simulink model "hw4_tank_PP"  (R2023b)
settings: Solver=ode45  StartTime=0.0  StopTime=50  FixedStep=0.000001  RelTol=1e-3
values from neighbouring files (symbols this model uses):
  A = 1    [Copy_of_hw1_four_channel_bilateral_teleoperation_params.m]    (also in hw1_four_channel_bilateral_teleoperation_params.m; hw2_2_3_channel_bilateral_teleoperation_params.m; hw3_scattering_teleop_FP_params.m = 1.5; hw3_scattering_teleop_PP_params.m)
  Ak = [1 Ts ... (first row only)    [hw3_scattering_teleop_FP_params.m]    (also in hw3_scattering_teleop_PP_params.m; hw4_tank_FP_params.m; hw4_tank_PP_params.m; no_noise_hw4_tank_PP_params.m)
  B = [Ts^2/2; Ts]    [hw3_scattering_teleop_FP_params.m]    (also in hw3_scattering_teleop_PP_params.m; hw4_tank_FP_params.m; hw4_tank_PP_params.m; no_noise_hw4_tank_PP_params.m)
  Be = 100    [Copy_of_hw1_four_channel_bilateral_teleoperation_params.m]    (also in hw1_four_channel_bilateral_teleoperation_params.m; hw2_2_3_channel_bilateral_teleoperation_params.m; hw3_scattering_teleop_FP_params.m; hw3_scattering_teleop_PP_params.m)
  beta = 0.1    [hw4_tank_FP_params.m]    (also in hw4_tank_PP_params.m; no_noise_hw4_tank_PP_params.m; test_no_noise_hw4_tank_PP_params.m)
  Bh = 1    [Copy_of_hw1_four_channel_bilateral_teleoperation_params.m]    (also in hw1_four_channel_bilateral_teleoperation_params.m; hw2_2_3_channel_bilateral_teleoperation_params.m; hw3_scattering_teleop_FP_params.m; hw3_scattering_teleop_PP_params.m)
  Bm = 20*0.8    (= 16)    [Copy_of_hw1_four_channel_bilateral_teleoperation_params.m]    (also in hw1_four_channel_bilateral_teleoperation_params.m; hw2_2_3_channel_bilateral_teleoperation_params.m; hw3_scattering_teleop_FP_params.m; hw3_scattering_teleop_PP_params.m)
  Bs = 4*Bm    (= 64)    [Copy_of_hw1_four_channel_bilateral_teleoperation_params.m]    (also in hw1_four_channel_bilateral_teleoperation_params.m; hw2_2_3_channel_bilateral_teleoperation_params.m; hw3_scattering_teleop_FP_params.m; hw3_scattering_teleop_PP_params.m)
  C = [1 0]    [hw3_scattering_teleop_FP_params.m]    (also in hw3_scattering_teleop_PP_params.m; hw4_tank_FP_params.m; hw4_tank_PP_params.m; no_noise_hw4_tank_PP_params.m)
  d = 1    [hw2_2_3_channel_bilateral_teleoperation_params.m]    (also in hw3_scattering_teleop_FP_params.m = 10; hw3_scattering_teleop_PP_params.m = 10; hw4_tank_FP_params.m = 10; hw4_tank_PP_params.m = 10)
  Dh = 20*0.8    (= 16)    [Copy_of_hw1_four_channel_bilateral_teleoperation_params.m]    (also in hw1_four_channel_bilateral_teleoperation_params.m; hw2_2_3_channel_bilateral_teleoperation_params.m; hw3_scattering_teleop_FP_params.m; hw3_scattering_teleop_PP_params.m)
  Dm = 5    [Copy_of_hw1_four_channel_bilateral_teleoperation_params.m]    (also in hw1_four_channel_bilateral_teleoperation_params.m; hw2_2_3_channel_bilateral_teleoperation_params.m; hw3_scattering_teleop_FP_params.m; hw3_scattering_teleop_PP_params.m = 0)
  Ds = 10    [Copy_of_hw1_four_channel_bilateral_teleoperation_params.m]    (also in hw1_four_channel_bilateral_teleoperation_params.m; hw2_2_3_channel_bilateral_teleoperation_params.m; hw3_scattering_teleop_FP_params.m = 0; hw3_scattering_teleop_PP_params.m = 0)
  Fc = 1    [Copy_of_hw1_four_channel_bilateral_teleoperation_params.m]    (also in hw1_four_channel_bilateral_teleoperation_params.m; hw2_2_3_channel_bilateral_teleoperation_params.m; hw3_scattering_teleop_FP_params.m; hw3_scattering_teleop_PP_params.m)
  Flp = 0.5    [Copy_of_hw1_four_channel_bilateral_teleoperation_params.m]    (also in hw1_four_channel_bilateral_teleoperation_params.m; hw2_2_3_channel_bilateral_teleoperation_params.m; hw3_scattering_teleop_FP_params.m = 0.01; hw3_scattering_teleop_PP_params.m = 0.01)
  Flp1 = 0.5    [hw3_scattering_teleop_FP_params.m]    (also in hw3_scattering_teleop_PP_params.m; hw4_tank_FP_params.m; hw4_tank_PP_params.m; no_noise_hw4_tank_PP_params.m)
  Hd = 1    [hw4_tank_FP_params.m]    (also in hw4_tank_PP_params.m; no_noise_hw4_tank_PP_params.m; test_no_noise_hw4_tank_PP_params.m)
  Hm_init = 5    [hw4_tank_FP_params.m]    (also in hw4_tank_PP_params.m; no_noise_hw4_tank_PP_params.m; test_no_noise_hw4_tank_PP_params.m = 0)
  Hs_init = 5    [hw4_tank_FP_params.m]    (also in hw4_tank_PP_params.m; no_noise_hw4_tank_PP_params.m; test_no_noise_hw4_tank_PP_params.m = 0)
  Jh = 1    [Copy_of_hw1_four_channel_bilateral_teleoperation_params.m]    (also in hw1_four_channel_bilateral_teleoperation_params.m; hw2_2_3_channel_bilateral_teleoperation_params.m; hw3_scattering_teleop_FP_params.m; hw3_scattering_teleop_PP_params.m)
  Ke = 200    [Copy_of_hw1_four_channel_bilateral_teleoperation_params.m]    (also in hw1_four_channel_bilateral_teleoperation_params.m; hw2_2_3_channel_bilateral_teleoperation_params.m; hw3_scattering_teleop_FP_params.m; hw3_scattering_teleop_PP_params.m)
  Km = 10*1    (= 10)    [Copy_of_hw1_four_channel_bilateral_teleoperation_params.m]    (also in hw1_four_channel_bilateral_teleoperation_params.m; hw2_2_3_channel_bilateral_teleoperation_params.m; hw3_scattering_teleop_FP_params.m; hw3_scattering_teleop_PP_params.m)
  Ks = 4*Km    (= 40)    [Copy_of_hw1_four_channel_bilateral_teleoperation_params.m]    (also in hw1_four_channel_bilateral_teleoperation_params.m; hw2_2_3_channel_bilateral_teleoperation_params.m; hw3_scattering_teleop_FP_params.m; hw3_scattering_teleop_PP_params.m)
  Mm = 0.5    [Copy_of_hw1_four_channel_bilateral_teleoperation_params.m]    (also in hw1_four_channel_bilateral_teleoperation_params.m; hw2_2_3_channel_bilateral_teleoperation_params.m; hw3_scattering_teleop_FP_params.m; hw3_scattering_teleop_PP_params.m)
  Ms = 2    [Copy_of_hw1_four_channel_bilateral_teleoperation_params.m]    (also in hw1_four_channel_bilateral_teleoperation_params.m; hw2_2_3_channel_bilateral_teleoperation_params.m; hw3_scattering_teleop_FP_params.m; hw3_scattering_teleop_PP_params.m)
  noise = 0.001    [hw3_scattering_teleop_FP_params.m]    (also in hw3_scattering_teleop_PP_params.m; hw4_tank_FP_params.m = 0.0001; hw4_tank_PP_params.m; no_noise_hw4_tank_PP_params.m)
  Ph = 10*1    (= 10)    [Copy_of_hw1_four_channel_bilateral_teleoperation_params.m]    (also in hw1_four_channel_bilateral_teleoperation_params.m; hw2_2_3_channel_bilateral_teleoperation_params.m; hw3_scattering_teleop_FP_params.m; hw3_scattering_teleop_PP_params.m)
  R = 1    [hw3_scattering_teleop_FP_params.m]    (also in hw3_scattering_teleop_PP_params.m; hw4_tank_FP_params.m; hw4_tank_PP_params.m; no_noise_hw4_tank_PP_params.m)
  tlcAlpha = 2    [hw4_tank_FP_params.m]    (also in hw4_tank_PP_params.m; no_noise_hw4_tank_PP_params.m; test_no_noise_hw4_tank_PP_params.m)
  Ts = 0.001    [hw3_scattering_teleop_FP_params.m]    (also in hw3_scattering_teleop_PP_params.m; hw4_tank_FP_params.m; hw4_tank_PP_params.m; no_noise_hw4_tank_PP_params.m)
  x0 = [0 0]    [hw3_scattering_teleop_FP_params.m]    (also in hw3_scattering_teleop_PP_params.m; hw4_tank_FP_params.m; hw4_tank_PP_params.m; no_noise_hw4_tank_PP_params.m)
  xe = 5    [Copy_of_hw1_four_channel_bilateral_teleoperation_params.m]    (also in hw1_four_channel_bilateral_teleoperation_params.m = 0.8; hw2_2_3_channel_bilateral_teleoperation_params.m = 2; hw3_scattering_teleop_FP_params.m = 0.8; hw3_scattering_teleop_PP_params.m = 2)
undefined symbols (not defined in the file or in its folder): Discrete, Time
libraries: simulink x3, ctrlSharedLib x2, cstblocks x1
settings Model: Creator=86180  LastModifiedBy=86180

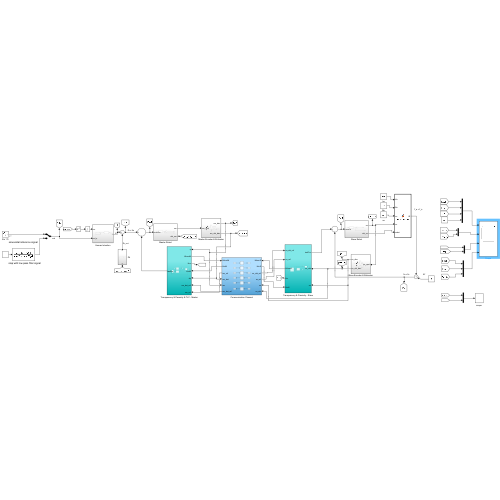
[thumbnail: Simulink's stored preview of the top-level diagram]
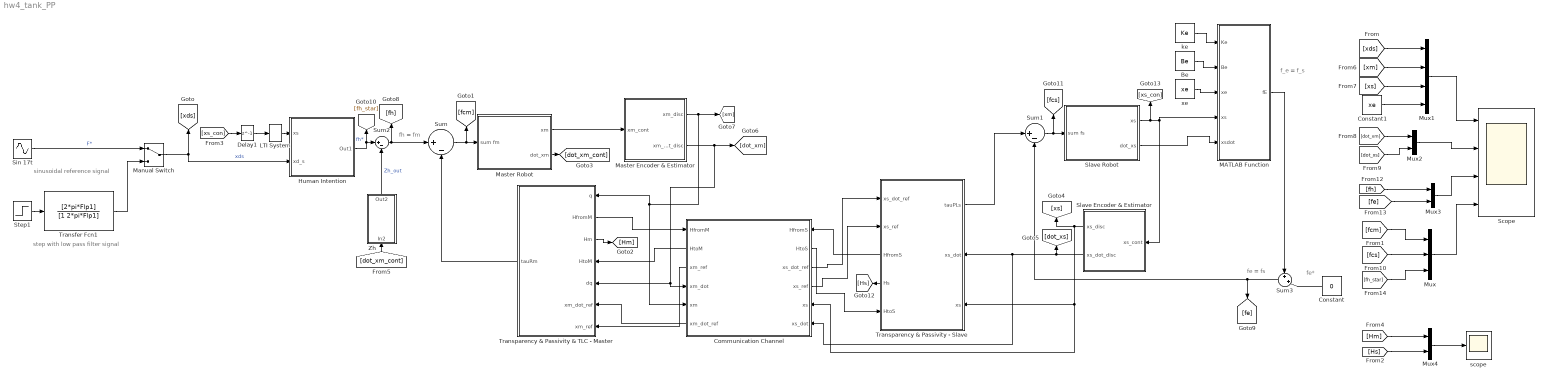
== system hw4_tank_PP ==
  note: f_e = f_s
  note: fe*
  note: fe = fs
  note: fh = fm
  note: sinusoidal reference signal
  note: step with low pass filter signal
  Be : Constant  Value=Be
  Communication Channel : Subsystem
      settings: PortSchema="{\"entries\":[{\"content\":{\"sides\":[{\"content\":{\"connectorIds\":[\"In1\",\"Out4\",\"Out5\",\"Out6\",\"In2\",\"In3\"]},\"type\":\"ConnectorPlacement.EquallySpacedRectSide\",\"uuid\":\"1c070cf8-9aa7-4f7b-8e2f-2632c2893f69\"},{\"content\":{\"connectorIds\":[\"In4\",\"Out1\",\"Out2\",\"In5\",\"In6\",\"Out3\"],\"side\":\"RIGHT\"},\"type\":\"ConnectorPlacement.EquallySpacedRectSide\",\"uuid\":\"32173565-3523-4dfc-9820-763c87098354\"},{\"content\":{\"side\":\"TOP\"},\"type\":\"ConnectorPlacement.EquallySpacedRectSide\",\"uuid\":\"13187df6-bf6f-436e-a2ee-34150977e6a8\"},{\"content\":{\"side\":\"HIDDEN\"},\"type\":\"ConnectorPlacement.EquallySpacedRectSide\",\"uuid\":\"1e5bcdd7-6028-40f7-b524-727817e519ff\"}]},\"type\":\"ConnectorPlacement.EquallySpacedConnector\",\"uuid\":\"c84d0440-83b9-4b92-a10a-1f72bb115b54\"}],\"packageUris\":[\"http://schema.mathworks.com/mf0/Connector/R2020b\"],\"version\":\"1.0\"}"
  Constant : Constant  Value=0
  Constant1 : Constant  Value=xe
  Delay1 : Delay  DelayLength=1  SampleTime=Ts
  Human Intention : Subsystem
  LTI System : cstblocks/LTI System  sys=1  IC=[]  PadeOrder=0
  MATLAB Function : MATLAB Function  TreatAsAtomicUnit=on
  Manual Switch : ManualSwitch
  Master Encoder & Estimator : Subsystem
  Master Robot : Subsystem
  Mux : Mux  Inputs=3
  Mux1 : Mux
  Mux2 : Mux  Inputs=2
  Mux3 : Mux  Inputs=2
  Mux4 : Mux  Inputs=2
  Scope : Scope  NumInputPorts=4
  Sin 17t : Sin  Amplitude=A  Frequency=Fc  SampleTime=0
  Slave Encoder & Estimator : Subsystem
  Slave Robot : Subsystem
  Step1 : Step  Time=0.5  After=A  SampleTime=0
  Sum : Sum  Inputs=|+-
  Sum1 : Sum  Inputs=|+-
  Sum2 : Sum  Inputs=|+-
  Sum3 : Sum  Inputs=+|+|
  Transfer Fcn1 : TransferFcn  Numerator=[2*pi*Flp1]  Denominator=[1 2*pi*Flp1]
  Transparency & Passivity & TLC - Master : Subsystem
      settings: PortSchema="{\"entries\":[{\"content\":{\"sides\":[{\"content\":{\"connectorIds\":[\"In1\",\"Out2\",\"Out3\",\"In2\",\"In3\",\"In4\",\"In5\"]},\"type\":\"ConnectorPlacement.EquallySpacedRectSide\",\"uuid\":\"254acbc8-8c2d-438f-adc1-7e75d47258bf\"},{\"content\":{\"connectorIds\":[\"Out1\"],\"side\":\"RIGHT\"},\"type\":\"ConnectorPlacement.EquallySpacedRectSide\",\"uuid\":\"ebc7579d-fe16-4fae-be7d-b1631322842e\"},{\"content\":{\"side\":\"TOP\"},\"type\":\"ConnectorPlacement.EquallySpacedRectSide\",\"uuid\":\"d0c6f2f9-df1e-40c2-885e-c029821bef96\"}]},\"type\":\"ConnectorPlacement.EquallySpacedConnector\",\"uuid\":\"8dee1f1f-c5e6-463a-a0e9-fbee882b1e3c\"}],\"packageUris\":[\"http://schema.mathworks.com/mf0/Connector/R2020b\"],\"version\":\"1.0\"}"
  Transparency & Passivity - Slave : Subsystem
      settings: PortSchema="{\"entries\":[{\"content\":{\"sides\":[{\"content\":{\"connectorIds\":[\"In1\",\"In2\",\"Out2\",\"Out3\",\"In3\"]},\"type\":\"ConnectorPlacement.EquallySpacedRectSide\",\"uuid\":\"bd42ff73-50dc-42d6-9dfb-d60369543bc9\"},{\"content\":{\"connectorIds\":[\"Out1\",\"In4\",\"In5\"],\"side\":\"RIGHT\"},\"type\":\"ConnectorPlacement.EquallySpacedRectSide\",\"uuid\":\"78e50b8f-eeac-432c-8eb4-27f06d4ce9eb\"},{\"content\":{\"side\":\"TOP\"},\"type\":\"ConnectorPlacement.EquallySpacedRectSide\",\"uuid\":\"9e8e9e88-d3ad-4c46-818b-4ad777acb646\"}]},\"type\":\"ConnectorPlacement.EquallySpacedConnector\",\"uuid\":\"6c4e05d2-6c15-4cd7-9da0-0c4b09a4ecbf\"}],\"packageUris\":[\"http://schema.mathworks.com/mf0/Connector/R2020b\"],\"version\":\"1.0\"}"
  Zh : Subsystem
  ke : Constant  Value=Ke
  scope : Scope
  xe : Constant  Value=xe
  wires:
  Manual Switch/1 -> Human Intention/2(xd_s), [xds]  "xds"
  Zh/1(Out2) -> Sum2/2  "Zh_out"
  Transfer Fcn1/1 -> Manual Switch/2
  Human Intention/1(Out1) -> [fh_star], Sum2/1  "fh*"
  Sin 17t/1 -> Manual Switch/1  "F*"
  Step1/1 -> Transfer Fcn1/1
  ke/1 -> MATLAB Function/1(Ke)
  xe/1 -> MATLAB Function/3(xe)
  Slave Robot/1(xs) -> MATLAB Function/4(xs), Slave Encoder & Estimator/1(xs_cont), [xs_con]
  MATLAB Function/1(fE) -> Sum3/1
  Be/1 -> MATLAB Function/2(Be)
  Sum2/1 -> Sum/1, [fh]
  Slave Robot/2(dot_xs) -> MATLAB Function/5(xsdot)
  Sum3/1 -> Sum1/2, [fe]
  Constant/1 -> Sum3/2
  [xds] -> Mux1/1
  Sum/1 -> [fcm], Master Robot/1(sum fm)
  [dot_xm_cont] -> Zh/1(In2)
  [xm] -> Mux1/2
  [xs] -> Mux1/3
  [dot_xm] -> Mux2/1
  Sum1/1 -> [fcs], Slave Robot/1(sum fs)
  [fh] -> Mux3/1
  [fe] -> Mux3/2
  [fh_star] -> Mux/3
  [fcs] -> Mux/2
  [fcm] -> Mux/1
  Constant1/1 -> Mux1/4
  [dot_xs] -> Mux2/2
  Mux1/1 -> Scope/1
  Mux2/1 -> Scope/2
  Mux3/1 -> Scope/3
  Mux/1 -> Scope/4
  [xs_con] -> Delay1/1
  Master Robot/1(xm) -> Master Encoder & Estimator/1(xm_cont)
  Master Encoder & Estimator/1(xm_disc) -> Communication Channel/6(xm), Transparency & Passivity & TLC - Master/1(q), [xm]
  Master Encoder & Estimator/2(xm_dot_disc) -> Communication Channel/5(xm_dot), Transparency & Passivity & TLC - Master/3(dq), [dot_xm]
  Slave Encoder & Estimator/2(xs_dot_disc) -> Communication Channel/3(xs_dot), Transparency & Passivity - Slave/4(xs_dot), [dot_xs]
  Slave Encoder & Estimator/1(xs_disc) -> Communication Channel/2(xs), Transparency & Passivity - Slave/5(xs), [xs]
  Delay1/1 -> LTI System/1
  LTI System/1 -> Human Intention/1(xs)
  Master Robot/2(dot_xm) -> [dot_xm_cont]
  Transparency & Passivity & TLC - Master/2(HfromM) -> Communication Channel/4(HfromM)
  Transparency & Passivity & TLC - Master/1(tauRm) -> Sum/2
  Communication Channel/1(HtoM) -> Transparency & Passivity & TLC - Master/2(HtoM)
  Transparency & Passivity - Slave/2(HfromS) -> Communication Channel/1(HfromS)
  Transparency & Passivity - Slave/1(tauPLs) -> Sum1/1
  Communication Channel/4(HtoS) -> Transparency & Passivity - Slave/3(HtoS)
  Communication Channel/5(xs_dot_ref) -> Transparency & Passivity - Slave/1(xs_dot_ref)
  Communication Channel/6(xs_ref) -> Transparency & Passivity - Slave/2(xs_ref)
  [Hm] -> Mux4/1
  [Hs] -> Mux4/2
  Mux4/1 -> scope/1
  Transparency & Passivity & TLC - Master/3(Hm) -> [Hm]
  Transparency & Passivity - Slave/3(Hs) -> [Hs]
  Communication Channel/2(xm_ref) -> Transparency & Passivity & TLC - Master/5(xm_ref)
  Communication Channel/3(xm_dot_ref) -> Transparency & Passivity & TLC - Master/4(xm_dot_ref)

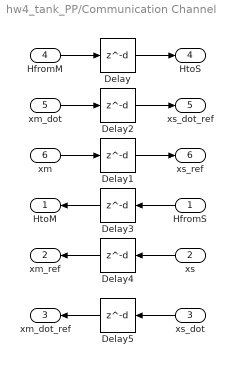
== system hw4_tank_PP/Communication Channel ==
  HfromS : Inport
  xs : Inport  Port=2
  xs_dot : Inport  Port=3
  HfromM : Inport  Port=4
  xm_dot : Inport  Port=5
  xm : Inport  Port=6
  Delay{,1..5} (6 alike) : Delay  DelayLength=d  SampleTime=Ts
  HtoM : Outport
  xm_ref : Outport  Port=2
  xm_dot_ref : Outport  Port=3
  HtoS : Outport  Port=4
  xs_dot_ref : Outport  Port=5
  xs_ref : Outport  Port=6
  wires:
  HfromS/1 -> Delay3/1
  xm_dot/1 -> Delay2/1
  xs/1 -> Delay4/1
  Delay4/1 -> xm_ref/1
  xm/1 -> Delay1/1
  Delay1/1 -> xs_ref/1
  Delay2/1 -> xs_dot_ref/1
  HfromM/1 -> Delay/1
  Delay/1 -> HtoS/1
  Delay3/1 -> HtoM/1
  Delay5/1 -> xm_dot_ref/1
  xs_dot/1 -> Delay5/1

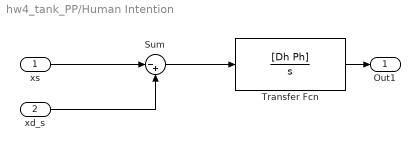
== system hw4_tank_PP/Human Intention ==
  xs : Inport
  xd_s : Inport  Port=2
  Sum : Sum  Inputs=|-+
  Transfer Fcn : TransferFcn  Numerator=[Dh Ph]  Denominator=[1 0]
  Out1 : Outport
  wires:
  Sum/1 -> Transfer Fcn/1
  xd_s/1 -> Sum/2
  xs/1 -> Sum/1
  Transfer Fcn/1 -> Out1/1

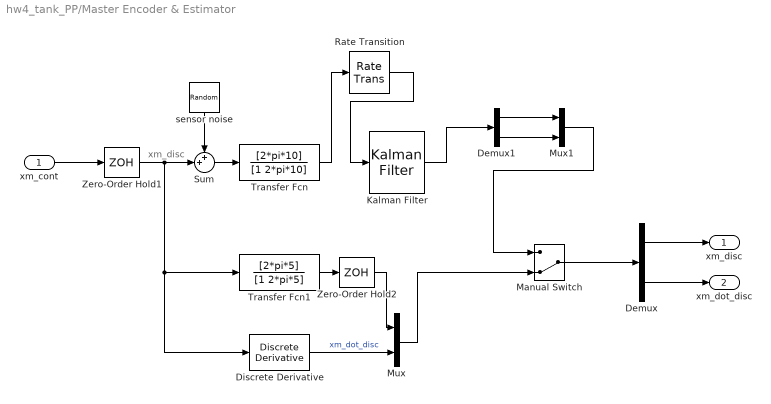
== system hw4_tank_PP/Master Encoder & Estimator ==
  note: xm_disc
  xm_cont : Inport
  Demux : Demux  Outputs=2
  Demux1 : Demux  Outputs=2
  Discrete Derivative : simulink/Discrete/Discrete Derivative  gainval=1.0  ICPrevScaledInput=0.0  OutMin=[]  OutMax=[]  OutDataType=fixdt(1, 16)  OutScaling=2^-10  DoSatur=off
  Kalman Filter : ctrlSharedLib/Kalman Filter  TimeDomain=Discrete-Time  UseCurrentEstimator=on  ModelSource=Individual A, B, C, D matrices  ModelSourceVariable=ss(0.95,1,1,0,1)  A=Ak  B=B  C=C  D=0  NumberOfStates=2  NumberOfInputs=1  NumberOfOutputs=1  InitialEstimateSource=Dialog  X0=x0  P0=10  UseK=off  UseGH=off  NumberOfProcessNoiseInputs=1  G=1  TimeInvariantG=on  H=0  TimeInvariantH=on  Q=Q_m  TimeInvariantQ=on  R=R  TimeInvariantR=on  N=0  TimeInvariantN=on  AddInputPort=off  AddEnablePort=off  OutputEstimatedY=off  OutputP=off  Ts=Ts
  Manual Switch : ManualSwitch  CurrentSetting=0
  Mux : Mux  Inputs=2
  Mux1 : Mux  Inputs=2
  Rate Transition : RateTransition
  Sum : Sum  Inputs=++|
  Transfer Fcn : TransferFcn  Numerator=[2*pi*10]  Denominator=[1 2*pi*10]
  Transfer Fcn1 : TransferFcn  Numerator=[2*pi*5]  Denominator=[1 2*pi*5]
  Zero-Order Hold1 : ZeroOrderHold  SampleTime=Ts
  Zero-Order Hold2 : ZeroOrderHold  SampleTime=Ts
  sensor noise : RandomNumber  Variance=noise  SampleTime=Ts
  xm_disc : Outport
  xm_dot_disc : Outport  Port=2
  wires:
  Demux/2 -> xm_dot_disc/1
  Discrete Derivative/1 -> Mux/2  "xm_dot_disc"
  Manual Switch/1 -> Demux/1
  Zero-Order Hold1/1 -> Discrete Derivative/1, Transfer Fcn1/1, Sum/2
  xm_cont/1 -> Zero-Order Hold1/1
  Demux/1 -> xm_disc/1
  sensor noise/1 -> Sum/1
  Mux/1 -> Manual Switch/2
  Mux1/1 -> Manual Switch/1
  Sum/1 -> Transfer Fcn/1
  Kalman Filter/1 -> Demux1/1
  Demux1/1 -> Mux1/1
  Demux1/2 -> Mux1/2
  Transfer Fcn/1 -> Rate Transition/1
  Rate Transition/1 -> Kalman Filter/1
  Transfer Fcn1/1 -> Zero-Order Hold2/1
  Zero-Order Hold2/1 -> Mux/1

== system hw4_tank_PP/Master Robot ==
  note: dot_xm
  note: xm
      | xm
  sum fm : Inport
  Integrator1 : Integrator
  Transfer Fcn : TransferFcn  Denominator=[Mm Dm]
  xm : Outport
  dot_xm : Outport  Port=2
  wires:
  Integrator1/1 -> xm/1
  Transfer Fcn/1 -> dot_xm/1, Integrator1/1
  sum fm/1 -> Transfer Fcn/1

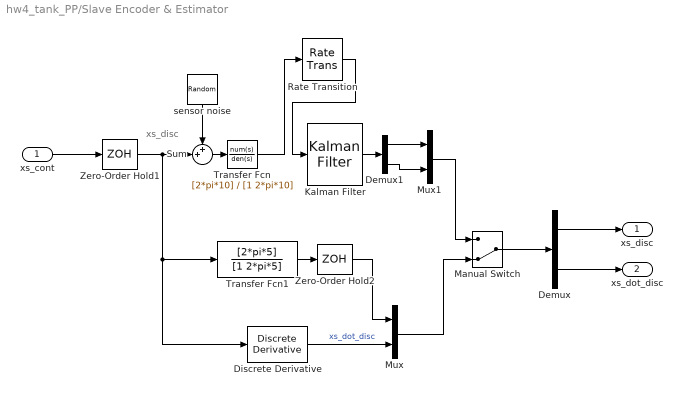
== system hw4_tank_PP/Slave Encoder & Estimator ==
  note: xs_disc
  xs_cont : Inport
  Demux : Demux  Outputs=2
  Demux1 : Demux  Outputs=2
  Discrete Derivative : simulink/Discrete/Discrete Derivative  gainval=1.0  ICPrevScaledInput=0.0  OutMin=[]  OutMax=[]  OutDataType=fixdt(1, 16)  OutScaling=2^-10  DoSatur=off
  Kalman Filter : ctrlSharedLib/Kalman Filter  TimeDomain=Discrete-Time  UseCurrentEstimator=on  ModelSource=Individual A, B, C, D matrices  ModelSourceVariable=ss(0.95,1,1,0,1)  A=Ak  B=B  C=C  D=0  NumberOfStates=2  NumberOfInputs=1  NumberOfOutputs=1  InitialEstimateSource=Dialog  X0=0  P0=10  UseK=off  UseGH=off  NumberOfProcessNoiseInputs=1  G=1  TimeInvariantG=on  H=0  TimeInvariantH=on  Q=Q_m  TimeInvariantQ=on  R=R  TimeInvariantR=on  N=0  TimeInvariantN=on  AddInputPort=off  AddEnablePort=off  OutputEstimatedY=off  OutputP=off  Ts=Ts
  Manual Switch : ManualSwitch  CurrentSetting=0
  Mux : Mux  Inputs=2
  Mux1 : Mux  Inputs=2
  Rate Transition : RateTransition
  Sum : Sum  Inputs=++|
  Transfer Fcn : TransferFcn  Numerator=[2*pi*10]  Denominator=[1 2*pi*10]
  Transfer Fcn1 : TransferFcn  Numerator=[2*pi*5]  Denominator=[1 2*pi*5]
  Zero-Order Hold1 : ZeroOrderHold  SampleTime=Ts
  Zero-Order Hold2 : ZeroOrderHold  SampleTime=Ts
  sensor noise : RandomNumber  Variance=noise  SampleTime=Ts
  xs_disc : Outport
  xs_dot_disc : Outport  Port=2
  wires:
  Demux/2 -> xs_dot_disc/1
  Discrete Derivative/1 -> Mux/2  "xs_dot_disc"
  Manual Switch/1 -> Demux/1
  xs_cont/1 -> Zero-Order Hold1/1
  Demux/1 -> xs_disc/1
  sensor noise/1 -> Sum/1
  Mux/1 -> Manual Switch/2
  Sum/1 -> Transfer Fcn/1
  Mux1/1 -> Manual Switch/1
  Kalman Filter/1 -> Demux1/1
  Demux1/1 -> Mux1/1
  Demux1/2 -> Mux1/2
  Transfer Fcn/1 -> Rate Transition/1
  Rate Transition/1 -> Kalman Filter/1
  Zero-Order Hold1/1 -> Discrete Derivative/1, Transfer Fcn1/1, Sum/2
  Transfer Fcn1/1 -> Zero-Order Hold2/1
  Zero-Order Hold2/1 -> Mux/1

== system hw4_tank_PP/Slave Robot ==
  note: dot_xs
  note: xs
      | xm
  sum fs : Inport
  Integrator1 : Integrator
  Transfer Fcn : TransferFcn  Denominator=[Ms Ds]
  xs : Outport
  dot_xs : Outport  Port=2
  wires:
  Integrator1/1 -> xs/1
  Transfer Fcn/1 -> dot_xs/1, Integrator1/1
  sum fs/1 -> Transfer Fcn/1

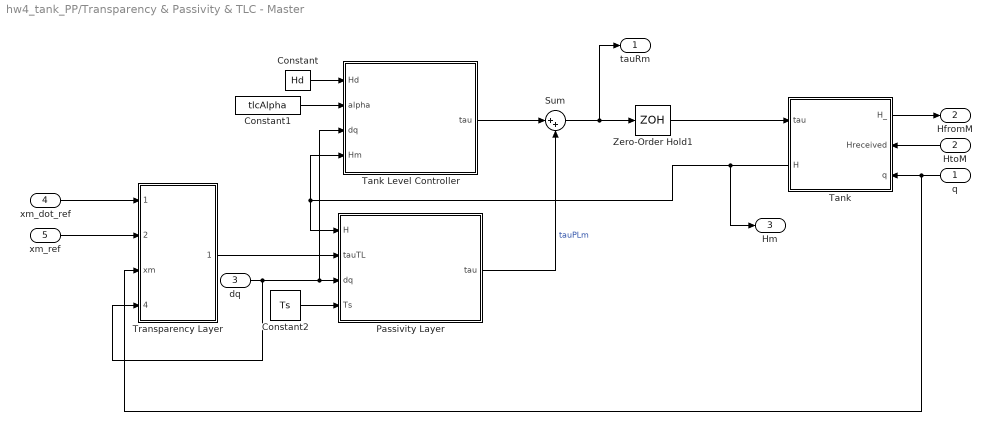
== system hw4_tank_PP/Transparency & Passivity & TLC - Master ==
  q : Inport
  HtoM : Inport  Port=2
  dq : Inport  Port=3
  xm_dot_ref : Inport  Port=4
  xm_ref : Inport  Port=5
  Constant : Constant  Value=Hd
  Constant1 : Constant  Value=tlcAlpha
  Constant2 : Constant  Value=Ts
  Passivity Layer : MATLAB Function  TreatAsAtomicUnit=on
  Sum : Sum  Inputs=|++
  Tank : Subsystem
      settings: PortSchema="{\"entries\":[{\"content\":{\"sides\":[{\"content\":{\"connectorIds\":[\"Out2\",\"In1\",\"In2\"]},\"type\":\"ConnectorPlacement.EquallySpacedRectSide\",\"uuid\":\"482b0a11-f044-49fa-a74d-4dac8b5b787b\"},{\"content\":{\"connectorIds\":[\"In3\",\"Out1\"],\"side\":\"RIGHT\"},\"type\":\"ConnectorPlacement.EquallySpacedRectSide\",\"uuid\":\"b0c369ed-ae40-43d8-b393-bca9f7720d62\"},{\"content\":{\"connectorIds\":[],\"side\":\"TOP\"},\"type\":\"ConnectorPlacement.EquallySpacedRectSide\",\"uuid\":\"ff021616-d6aa-4c0a-874b-a9ebe947c92c\"},{\"content\":{\"connectorIds\":[],\"side\":\"BOTTOM\"},\"type\":\"ConnectorPlacement.EquallySpacedRectSide\",\"uuid\":\"4e18ee96-bca7-41b6-9abb-5b593b41c296\"},{\"content\":{\"connectorIds\":[],\"side\":\"HIDDEN\"},\"type\":\"ConnectorPlacement.EquallySpacedRectSide\",\"uuid\":\"be815b34-35c7-4c6f-8c8b-4a812b3d12e9\"}]},\"type\":\"ConnectorPlacement.EquallySpacedConnector\",\"uuid\":\"78552b8a-5f1c-4815-a807-de98f58b7f2e\"}],\"packageUris\":[\"http://schema.mathworks.com/mf0/Connector/R2020b\"],\"version\":\"1.0\"}"
  Tank Level Controller : MATLAB Function  TreatAsAtomicUnit=on
  Transparency Layer : Subsystem
  Zero-Order Hold1 : ZeroOrderHold  SampleTime=Ts
  tauRm : Outport
  HfromM : Outport  Port=2
  Hm : Outport  Port=3
  wires:
  Tank Level Controller/1(tau) -> Sum/1
  Passivity Layer/1(tau) -> Sum/2  "tauPLm"
  Zero-Order Hold1/1 -> Tank/3(tau)
  Tank/1(H) -> Hm/1, Passivity Layer/1(H), Tank Level Controller/4(Hm)
  dq/1 -> Transparency Layer/4(xm_dot), Tank Level Controller/3(dq), Passivity Layer/3(dq)
  Constant2/1 -> Passivity Layer/4(Ts)
  Tank/2(H_) -> HfromM/1
  Constant/1 -> Tank Level Controller/1(Hd)
  Constant1/1 -> Tank Level Controller/2(alpha)
  Sum/1 -> tauRm/1, Zero-Order Hold1/1
  q/1 -> Transparency Layer/3(xm), Tank/2(q)
  HtoM/1 -> Tank/1(Hreceived)
  Transparency Layer/1(tauTLm) -> Passivity Layer/2(tauTL)
  xm_dot_ref/1 -> Transparency Layer/1(xm_dot_cmd)
  xm_ref/1 -> Transparency Layer/2(xm_cmd)

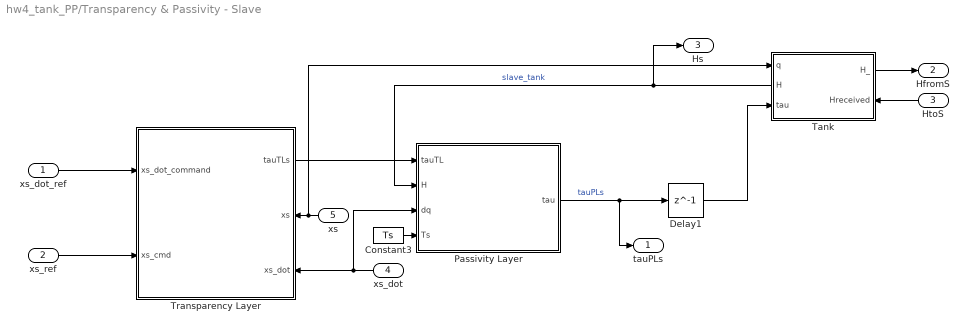
== system hw4_tank_PP/Transparency & Passivity - Slave ==
  xs_dot_ref : Inport
  xs_ref : Inport  Port=2
  HtoS : Inport  Port=3
  xs_dot : Inport  Port=4
  xs : Inport  Port=5
  Constant3 : Constant  Value=Ts
  Delay1 : Delay  DelayLength=1  SampleTime=Ts
  Passivity Layer : MATLAB Function  TreatAsAtomicUnit=on
  Tank : Subsystem
      settings: PortSchema="{\"entries\":[{\"content\":{\"sides\":[{\"content\":{\"connectorIds\":[\"In1\",\"Out2\",\"In2\"]},\"type\":\"ConnectorPlacement.EquallySpacedRectSide\",\"uuid\":\"482b0a11-f044-49fa-a74d-4dac8b5b787b\"},{\"content\":{\"connectorIds\":[\"Out1\",\"In3\"],\"side\":\"RIGHT\"},\"type\":\"ConnectorPlacement.EquallySpacedRectSide\",\"uuid\":\"b0c369ed-ae40-43d8-b393-bca9f7720d62\"},{\"content\":{\"connectorIds\":[],\"side\":\"TOP\"},\"type\":\"ConnectorPlacement.EquallySpacedRectSide\",\"uuid\":\"ff021616-d6aa-4c0a-874b-a9ebe947c92c\"},{\"content\":{\"connectorIds\":[],\"side\":\"BOTTOM\"},\"type\":\"ConnectorPlacement.EquallySpacedRectSide\",\"uuid\":\"4e18ee96-bca7-41b6-9abb-5b593b41c296\"},{\"content\":{\"connectorIds\":[],\"side\":\"HIDDEN\"},\"type\":\"ConnectorPlacement.EquallySpacedRectSide\",\"uuid\":\"be815b34-35c7-4c6f-8c8b-4a812b3d12e9\"}]},\"type\":\"ConnectorPlacement.EquallySpacedConnector\",\"uuid\":\"78552b8a-5f1c-4815-a807-de98f58b7f2e\"}],\"packageUris\":[\"http://schema.mathworks.com/mf0/Connector/R2020b\"],\"version\":\"1.0\"}"
  Transparency Layer : Subsystem
      settings: PortSchema="{\"entries\":[{\"content\":{\"sides\":[{\"content\":{\"connectorIds\":[\"In1\",\"In2\"]},\"type\":\"ConnectorPlacement.EquallySpacedRectSide\",\"uuid\":\"c8f256d1-8287-4bc6-9264-40c0684f6acd\"},{\"content\":{\"connectorIds\":[\"Out1\",\"In3\",\"In4\"],\"side\":\"RIGHT\"},\"type\":\"ConnectorPlacement.EquallySpacedRectSide\",\"uuid\":\"cb9f571e-93fc-426e-a4f2-aa96ae3bd6b3\"},{\"content\":{\"connectorIds\":[],\"side\":\"TOP\"},\"type\":\"ConnectorPlacement.EquallySpacedRectSide\",\"uuid\":\"b9b91304-f20e-4a66-aa64-b99c686ee85a\"},{\"content\":{\"connectorIds\":[],\"side\":\"HIDDEN\"},\"type\":\"ConnectorPlacement.EquallySpacedRectSide\",\"uuid\":\"c3abcf5a-e3b9-4b9a-a4b1-68c5725be1f4\"}]},\"type\":\"ConnectorPlacement.EquallySpacedConnector\",\"uuid\":\"83907002-acbd-4948-aeba-a43201e13c19\"}],\"packageUris\":[\"http://schema.mathworks.com/mf0/Connector/R2020b\"],\"version\":\"1.0\"}"
  tauPLs : Outport
  HfromS : Outport  Port=2
  Hs : Outport  Port=3
  wires:
  xs_dot_ref/1 -> Transparency Layer/1(xs_dot_command)
  xs_ref/1 -> Transparency Layer/2(xs_cmd)
  Transparency Layer/1(tauTLs) -> Passivity Layer/1(tauTL)
  xs/1 -> Tank/1(q), Transparency Layer/3(xs)
  Constant3/1 -> Passivity Layer/4(Ts)
  xs_dot/1 -> Passivity Layer/3(dq), Transparency Layer/4(xs_dot)
  Tank/2(H) -> Hs/1, Passivity Layer/2(H)  "slave_tank"
  Passivity Layer/1(tau) -> tauPLs/1, Delay1/1  "tauPLs"
  Delay1/1 -> Tank/2(tau)
  Tank/1(H_) -> HfromS/1
  HtoS/1 -> Tank/3(Hreceived)

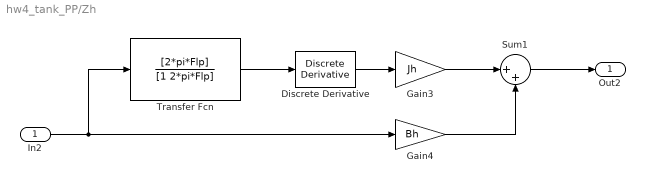
== system hw4_tank_PP/Zh ==
  In2 : Inport
  Discrete Derivative : simulink/Discrete/Discrete Derivative  gainval=1.0  ICPrevScaledInput=0.0  OutMin=[]  OutMax=[]  OutDataType=fixdt(1, 16)  OutScaling=2^-10  DoSatur=off
  Gain3 : Gain  Gain=Jh
  Gain4 : Gain  Gain=Bh
  Sum1 : Sum  Inputs=|++
  Transfer Fcn : TransferFcn  Numerator=[2*pi*Flp]  Denominator=[1 2*pi*Flp]
  Out2 : Outport
  wires:
  Gain3/1 -> Sum1/1
  In2/1 -> Transfer Fcn/1, Gain4/1
  Gain4/1 -> Sum1/2
  Transfer Fcn/1 -> Discrete Derivative/1
  Discrete Derivative/1 -> Gain3/1
  Sum1/1 -> Out2/1

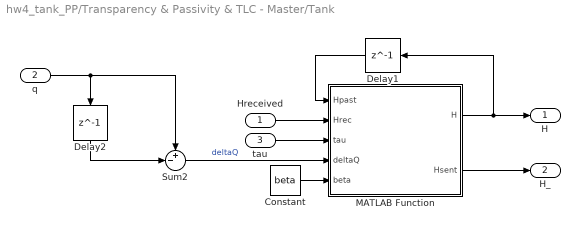
== system hw4_tank_PP/Transparency & Passivity & TLC - Master/Tank ==
  Hreceived : Inport
  q : Inport  Port=2
  tau : Inport  Port=3
  Constant : Constant  Value=beta
  Delay1 : Delay  DelayLength=1  InitialCondition=Hm_init  SampleTime=Ts
  Delay2 : Delay  DelayLength=1  SampleTime=Ts
  MATLAB Function : MATLAB Function  TreatAsAtomicUnit=on
  Sum2 : Sum  Inputs=+-|
  H : Outport
  H_ : Outport  Port=2
  wires:
  Delay2/1 -> Sum2/2
  q/1 -> Sum2/1, Delay2/1
  MATLAB Function/2(Hsent) -> H_/1
  Constant/1 -> MATLAB Function/5(beta)
  Sum2/1 -> MATLAB Function/4(deltaQ)  "deltaQ"
  Hreceived/1 -> MATLAB Function/2(Hrec)
  tau/1 -> MATLAB Function/3(tau)
  MATLAB Function/1(H) -> Delay1/1, H/1
  Delay1/1 -> MATLAB Function/1(Hpast)

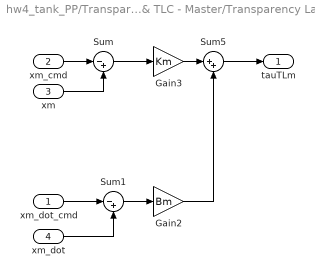
== system hw4_tank_PP/Transparency & Passivity & TLC - Master/Transparency Layer ==
  xm_dot_cmd : Inport
  xm_cmd : Inport  Port=2
  xm : Inport  Port=3
  xm_dot : Inport  Port=4
  Gain2 : Gain  Gain=Bm
  Gain3 : Gain  Gain=Km
  Sum : Sum  Inputs=|-+
  Sum1 : Sum  Inputs=|-+
  Sum5 : Sum  Inputs=|++
  tauTLm : Outport
  wires:
  Sum5/1 -> tauTLm/1
  Sum/1 -> Gain3/1
  Sum1/1 -> Gain2/1
  xm_dot_cmd/1 -> Sum1/1
  xm/1 -> Sum/2
  xm_dot/1 -> Sum1/2
  xm_cmd/1 -> Sum/1
  Gain3/1 -> Sum5/1
  Gain2/1 -> Sum5/2

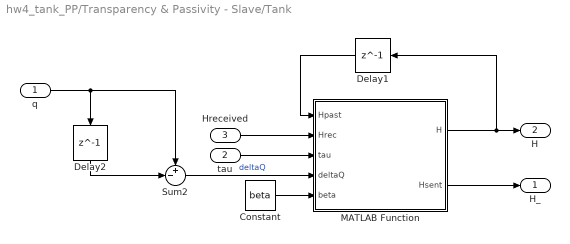
== system hw4_tank_PP/Transparency & Passivity - Slave/Tank ==
  q : Inport
  tau : Inport  Port=2
  Hreceived : Inport  Port=3
  Constant : Constant  Value=beta
  Delay1 : Delay  DelayLength=1  InitialCondition=Hs_init  SampleTime=Ts
  Delay2 : Delay  DelayLength=1  SampleTime=Ts
  MATLAB Function : MATLAB Function  TreatAsAtomicUnit=on
  Sum2 : Sum  Inputs=+-|
  H_ : Outport
  H : Outport  Port=2
  wires:
  Delay2/1 -> Sum2/2
  q/1 -> Sum2/1, Delay2/1
  MATLAB Function/2(Hsent) -> H_/1
  Constant/1 -> MATLAB Function/5(beta)
  Sum2/1 -> MATLAB Function/4(deltaQ)  "deltaQ"
  Hreceived/1 -> MATLAB Function/2(Hrec)
  tau/1 -> MATLAB Function/3(tau)
  MATLAB Function/1(H) -> Delay1/1, H/1
  Delay1/1 -> MATLAB Function/1(Hpast)

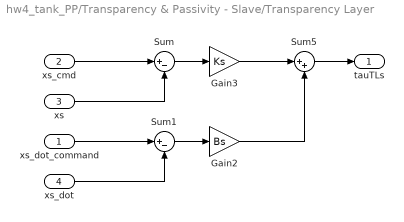
== system hw4_tank_PP/Transparency & Passivity - Slave/Transparency Layer ==
  xs_dot_command : Inport
  xs_cmd : Inport  Port=2
  xs : Inport  Port=3
  xs_dot : Inport  Port=4
  Gain2 : Gain  Gain=Bs
  Gain3 : Gain  Gain=Ks
  Sum : Sum  Inputs=|+-
  Sum1 : Sum  Inputs=|+-
  Sum5 : Sum  Inputs=|++
  tauTLs : Outport
  wires:
  Sum5/1 -> tauTLs/1
  xs/1 -> Sum/2
  xs_dot/1 -> Sum1/2
  xs_cmd/1 -> Sum/1
  xs_dot_command/1 -> Sum1/1
  Sum/1 -> Gain3/1
  Sum1/1 -> Gain2/1
  Gain3/1 -> Sum5/1
  Gain2/1 -> Sum5/2

== matlab function hw4_tank_PP/Transparency & Passivity & TLC - Master/Tank/MATLAB Function ==
  data: Hpast input; H output; Hrec input; tau input; deltaQ input; beta input; Hsent output
function [H,Hsent] = tank(Hpast, Hrec, tau, deltaQ, beta)
Hused = tau*deltaQ; % Slide 14
H = Hpast+Hrec-Hused; % Slide 16
Hsent = H*beta; % 
H = H-Hsent; % H k+1 % Slide 16

== matlab function hw4_tank_PP/MATLAB Function ==
  data: Ke input; fE output; Be input; xe input; xs input; xsdot input
function fE = environment(Ke, Be, xe, xs, xsdot)
    if xs > xe
        fE = Ke * (xs - xe) + Be * max(xsdot, 0); % Plot both contributions Ke and Be
    else
        fE = 0;
    end
end

== matlab function hw4_tank_PP/Transparency & Passivity & TLC - Master/Tank Level Controller ==
  data: Hd input; alpha input; dq input; tau output; Hm input
function tau = TLC(Hd,alpha,dq,Hm)
% Slide 20
if Hd <= Hm
    d = 0;
else
    d = alpha*(Hd-Hm);
end
tau = -d*dq;

== matlab function hw4_tank_PP/Transparency & Passivity - Slave/Passivity Layer ==
  data: tauTL input; H input; tau output; dq input; Ts input
function tau = tauPL(tauTL, H, dq,Ts)
% Slide 23
if H<= 0
    tauMax1 = 0;
else
    tauMax1 = tauTL;
end
tauMax2 = H/(dq*Ts);

tau = sign(tauTL)*min([abs(tauMax1),abs(tauMax2)]);

== matlab function hw4_tank_PP/Transparency & Passivity & TLC - Master/Passivity Layer ==
  data: H input; tauTL input; dq input; Ts input; tau output
function tau = PL(H,tauTL,dq,Ts)
% Slide 23
if H<= 0
    tauMax1 = 0;
else
    tauMax1 = tauTL;
end
tauMax2 = H/(dq*Ts);

tau = sign(tauTL)*min([abs(tauMax1),abs(tauMax2)]);

== matlab function hw4_tank_PP/Transparency & Passivity - Slave/Tank/MATLAB Function ==
  data: Hpast input; H output; Hrec input; tau input; deltaQ input; beta input; Hsent output
function [H,Hsent] = tank(Hpast, Hrec, tau, deltaQ, beta)
Hused = tau*deltaQ;% Slide 14
H = Hpast+Hrec-Hused; % Slide 16
Hsent = H*beta; %
H = H-Hsent; % H k+1 % Slide 16
